simulink model "model5"  (R2019b)
settings: Solver=VariableStepAuto  StartTime=0.0  StopTime=0.3  RelTol=1e-3
libraries: simulink x2
settings Model: Creator=surtweig  LastModifiedBy=surtweig

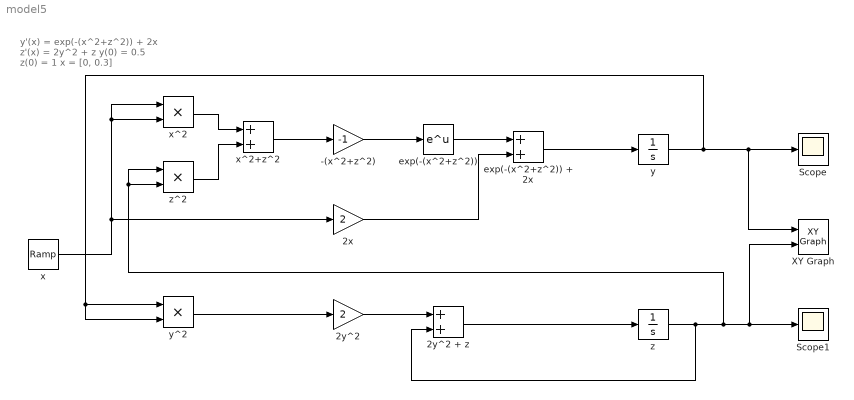
== system model5 ==
  note: y'(x) = exp(-(x^2+z^2)) + 2x
      | z'(x) = 2y^2 + z
      | y(0) = 0.5
      | z(0) = 1
      | x = [0, 0.3]
  -(x^2+z^2) : Gain  Gain=-1
  2x : Gain  Gain=2
  2y^2 : Gain  Gain=2
  2y^2 + z : Sum
  Scope : Scope
  Scope1 : Scope
  XY Graph : simulink/Sinks/XY Graph  xmin=-1  xmax=1  ymin=-1  ymax=1  st=-1
  exp(-(x^2+z^2)) : Math  SignedPower=off  SaturateOnIntegerOverflow=on
  exp(-(x^2+z^2)) + 2x : Sum
  x : simulink/Sources/Ramp  slope=1  start=0  InitialOutput=0
  x^2 : Product
  x^2+z^2 : Sum
  y : Integrator  InitialCondition=0.5
  y^2 : Product
  z : Integrator  InitialCondition=1
  z^2 : Product
  wires:
  -(x^2+z^2)/1 -> exp(-(x^2+z^2))/1
  x^2+z^2/1 -> -(x^2+z^2)/1
  exp(-(x^2+z^2))/1 -> exp(-(x^2+z^2)) + 2x/1
  2x/1 -> exp(-(x^2+z^2)) + 2x/2
  x^2/1 -> x^2+z^2/1
  z^2/1 -> x^2+z^2/2
  exp(-(x^2+z^2)) + 2x/1 -> y/1
  x/1 -> 2x/1, x^2/2, x^2/1
  2y^2 + z/1 -> z/1
  2y^2/1 -> 2y^2 + z/1
  y^2/1 -> 2y^2/1
  z/1 -> 2y^2 + z/2, z^2/1, z^2/2, XY Graph/2, Scope1/1
  y/1 -> y^2/2, y^2/1, XY Graph/1, Scope/1
